simulink model "theta_vp"  (R2024a)
settings: Solver=VariableStepAuto  StartTime=0.0  StopTime=10  RelTol=1e-3
values from neighbouring files (symbols this model uses):
  den_thetaVp = [Jeq*Lm / (Kt*N), Jeq*Rm / (Kt*N), Kb*N, 0]    [Hw2.m]
  Ks = 0.7990    (= 0.799)    [Hw2.m]
  num_thetaVp = [-1]    [Hw2.m]
settings Model: Creator=dunni  LastModifiedBy=dunni

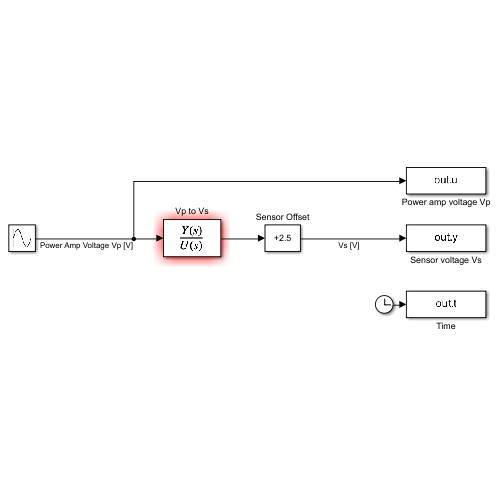
[thumbnail: Simulink's stored preview of the top-level diagram]
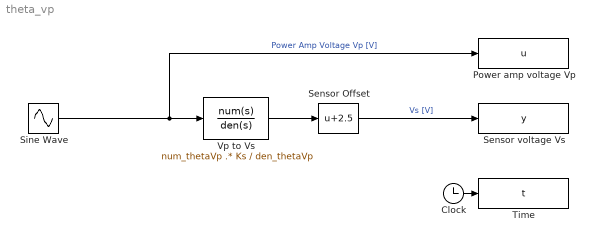
== system theta_vp ==
  Clock : Clock
  Power amp voltage Vp : ToWorkspace  VariableName=u  SampleTime=-1
  Sensor Offset : Bias  Bias=2.5  SaturateOnIntegerOverflow=off
  Sensor voltage Vs : ToWorkspace  VariableName=y  SampleTime=-1
  Sine Wave : Sin  Frequency=2*pi  SampleTime=0
  Time : ToWorkspace  VariableName=t  SampleTime=-1
  Vp to Vs : TransferFcn  Numerator=num_thetaVp .* Ks  Denominator=den_thetaVp
  wires:
  Sine Wave/1 -> Power amp voltage Vp/1, Vp to Vs/1  "Power Amp Voltage Vp [V]"
  Clock/1 -> Time/1
  Vp to Vs/1 -> Sensor Offset/1
  Sensor Offset/1 -> Sensor voltage Vs/1  "Vs [V]"
